simulink model "offlineDTOptim"  (R2019b)
settings: Solver=FixedStepAuto  StartTime=0.0  StopTime=tsim  FixedStep=1  MaxStep=1e-3  RelTol=1e-3  AbsTol=1e-3
PreLoadFcn:
  | coef = 220e-6; % Seebeck coefficient
  | R_int = 0.02; % Total electrical resistance
  | K = 1.5e-3; % Thermal conductance
  | T = 323.15; % Cold side temperature
  | 
  | 
StopFcn:
  | ee_addSimlogTimeStamp(bdroot)
values from neighbouring files (symbols this model uses):
  R = 3.3    [readSLDOData.m]
libraries: fl_lib x17, nesl_utility x10, ee_lib x5, simulink x2
CloseFcn:
  | try,close(h1_ee_peltier_device),end
  | clear h1_ee_peltier_device
  | 
  | clear simlog_ee_peltier_device
  | clear logsout_ee_peltier_device
  | clear COP_vec DT K R_int T coef j legend_data power simlog_Qc simlog_handles simlog_i simlog_v simout temp_cold_vec temp_hot temp_hot_vec
Description:
  | Use of Peltier Device as Thermoelectric Cooler
settings Model: OrderedModelArguments=off  Creator=The MathWorks, Inc.  LastModifiedBy=jairo
settings SolverCC: DecoupledContinuousIntegration=on
settings DataIOCC: SaveFormat=Array  ReturnWorkspaceOutputs=off  ReturnWorkspaceOutputsName=simout
settings OptimizationCC: LifeSpan=inf
settings DebuggingCC: UnderspecifiedInitializationDetection=Classic  MergeDetectMultiDrivingBlocksExec=none  SolverPrmCheckMsg=warning  FrameProcessingCompatibilityMsg=warning  StateNameClashWarn=warning  StrictBusMsg=ErrorOnBusTreatedAsVector  NonBusSignalsTreatedAsBus=error  SFUnexpectedBacktrackingDiag=warning  SFNoUnconditionalDefaultTransitionDiag=warning  ArithmeticOperatorsInVariantConditions=warning
settings HardwareCC: ProdBitPerPointer=32  ProdBitPerSizeT=32  ProdBitPerPtrDiffT=32  ProdLargestAtomicFloat=None  ProdIntDivRoundTo=Undefined  ProdEndianess=Unspecified  ProdWordSize=32  ProdHWDeviceType=32-bit Generic
settings ModelReferenceCC: PropagateSignalLabelsOutOfModel=off
settings SFSimCC: SimUseLocalCustomCode=off  CustomCodeUndefinedFunction=UseInterfaceOnly
settings RTWCC: RTWUseLocalCustomCode=off
settings GRTTargetCC: CodeReplacementLibrary=ANSI_C
settings SimscapeCC: SimscapeLogType=all  SimscapeLogSimulationStatistics=on  SimscapeLogName=simlog_ee_peltier_device  SimscapeLogDataHistory=10000

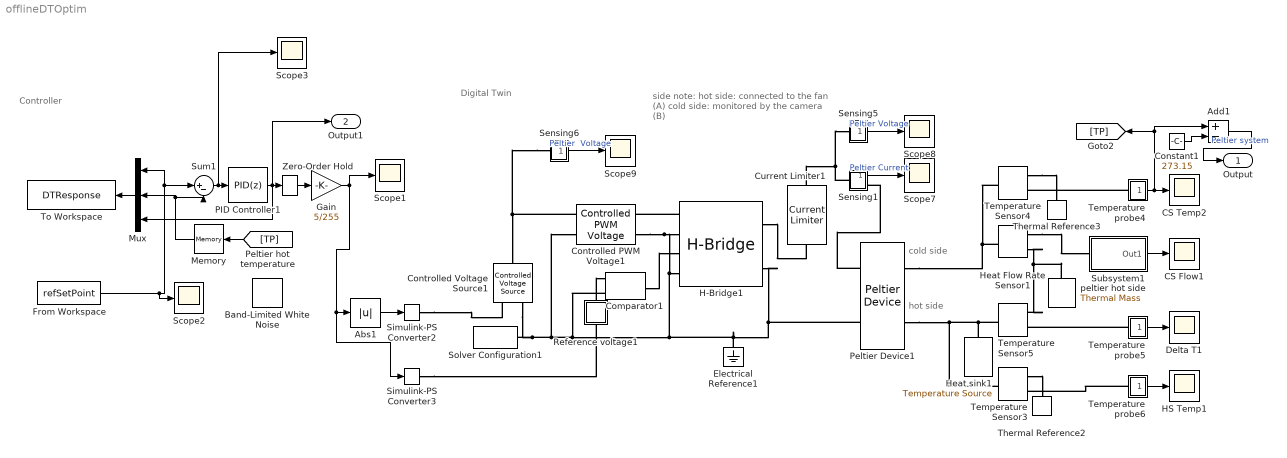
== system offlineDTOptim ==
  note: Digital Twin
  note: side note:
      |
      | hot side: connected to the fan (A)
      |
      | cold side: monitored by the camera (B)
  note: Controller
  note: cold side
  note: hot side
  Abs1 : Abs
  Add1 : Sum  Inputs=+-
  Band-Limited White Noise : simulink/Sources/Band-Limited White Noise  Cov=[0.005]  Ts=1  seed=[23341]
  CS Flow1 : Scope
  CS Temp2 : Scope
  Comparator1 : ee_lib/Integrated Circuits/Comparator  V_OS=5 mV  V_OL=0 V  V_OH=5 V  C_IN=0 pF  R_OUT=50 Ohm  Delay=0 s
      settings: SourceProductName=Simscape Electrical  SourceProductBaseCode=PS  InternalSimscapePortConfiguration="{\"Bottom\":[],\"Left\":[{\"id\":\"p\",\"label\":\"+\",\"type\":\"foundation.electrical.electrical\"},{\"id\":\"n\",\"label\":\"-\",\"type\":\"foundation.electrical.electrical\"}],\"Right\":[{\"id\":\"J\",\"label\":\"\",\"type\":\"foundation.electrical.electrical\"}],\"Top\":[]}"
  Constant1 : Constant  Value=273.15
  Controlled PWM Voltage1 : ee_lib/Integrated Circuits/Controlled PWM Voltage  F=4000 Hz  TD=0 s  pulse_width_offset=0 s  pulse_min=0 s  Vmin=0 V  Vmax=5 V  Vm=5 V  pwm_or_av=2  event_type=1  sample_time=5e-6 s  u_min=0  u_max=1
      settings: SourceProductName=Simscape Electrical
  Controlled Voltage Source1 : fl_lib/Electrical/Electrical Sources/Controlled Voltage Source
  Current Limiter1 : ee_lib/Semiconductors & Converters/Current Limiter  iLim=5 A  vLim=0.1 V  gLim=1e-3 1/Ohm  thermal_mass=100 J/K  initial_temperature=298.15 K
      settings: SourceProductName=Simscape Electrical  SourceProductBaseCode=PS  InternalSimscapePortConfiguration="{\"Bottom\":[],\"Left\":[{\"id\":\"p\",\"label\":\"+\",\"type\":\"foundation.electrical.electrical\"}],\"Right\":[{\"id\":\"n\",\"label\":\"-\",\"type\":\"foundation.electrical.electrical\"}],\"Top\":[]}"
  Delta T1 : Scope
  Electrical Reference1 : fl_lib/Electrical/Electrical Elements/Electrical Reference
  From Workspace : FromWorkspace  VariableName=refSetPoint  SampleTime=0
  Gain : Gain  Gain=5/255
  H-Bridge1 : ee_lib/Semiconductors & Converters/Converters/H-Bridge  supply_ports=ee.enum.supply_ports.hidesupply  Venable=2.5 V  Vmax=5 V  Vreverse=0.1 V  Vbrake=2.5 V  Vm=12 V  pwm_or_av=ee.enum.pwm_or_av.averaged  regenerative_braking_mode=ee.enum.converters.regenerative_braking_mode.always_enabled  discontinuous=ee.enum.current_profile.continuous  freewheeling_mode=ee.enum.converters.freewheeling_mode.one_switch_one_diode  Ron=0.1 Ohm  Don=0.1 Ohm  Goff=1e-6 S  Rload=3.38+0.1 Ohm  Lload=1e-5 H  F=4 kHz  thermal_mass=100 J/K  initial_temperature=298.15 K  Ron2=0.1 Ohm  Don2=0.05 Ohm  Tmeas=298.15 K  Tmeas2=398.15 K
      settings: SourceProductName=Simscape Electrical
  HS Temp1 : Scope
  Heat Flow Rate Sensor1 : fl_lib/Thermal/Thermal Sensors/Heat Flow Rate Sensor
      settings: SourceProductName=Simscape  SourceProductBaseCode=SS
  Heat sink1 : fl_lib/Thermal/Thermal Sources/Temperature Source  temperature=296 K
      settings: SourceProductName=Simscape
  Memory : Memory  InitialCondition=295
  Mux : Mux  Inputs=3
  PID Controller1 : simulink/Continuous/PID Controller  Controller=PID  Form=Parallel  TimeDomain=Discrete-time  SampleTime=1  IntegratorMethod=Forward Euler  FilterMethod=Forward Euler  ControllerParametersSource=internal  P=38.57  I=1.46877  D=6.66875  UseFilter=off  N=100  TunerSelectOption=Transfer Function Based (PID Tuner App)  InitialConditionSource=internal  InitialConditionForIntegrator=0  InitialConditionForFilter=0  DifferentiatorICPrevScaledInput=0  ExternalReset=none  TrackingMode=off  Kt=1  LimitOutput=on  UpperSaturationLimit=255  LowerSaturationLimit=-255  LinearizeAsGain=on  AntiWindupMode=back-calculation  Kb=1  POutMin=[]  POutMax=[]  IOutMin=[]  IOutMax=[]  DOutMin=[]  DOutMax=[]  NOutMin=[]  NOutMax=[]  SumOutMin=[]  SumOutMax=[]  SaturationOutMin=[]  SaturationOutMax=[]  PParamMin=[]  PParamMax=[]  IParamMin=[]  IParamMax=[]  DParamMin=[]  DParamMax=[]  NParamMin=[]  NParamMax=[]  KbParamMin=[]  KbParamMax=[]  KtParamMin=[]  KtParamMax=[]  KbOutMin=[]  KbOutMax=[]  KtOutMin=[]  KtOutMax=[]  IntegratorOutMin=[]  IntegratorOutMax=[]  FilterOutMin=[]  FilterOutMax=[]  SumI1OutMin=[]  SumI1OutMax=[]  SumI2OutMin=[]  SumI2OutMax=[]  SumI3OutMin=[]  SumI3OutMax=[]  SumI4OutMin=[]  SumI4OutMax=[]  SumDOutMin=[]  SumDOutMax=[]  DifferentiatorOutMin=[]  DifferentiatorOutMax=[]  FilterDiffOutCoefMin=[]  FilterDiffOutCoefMax=[]  ReciprocalOutMin=[]  ReciprocalOutMax=[]  SumDenOutMin=[]  SumDenOutMax=[]  SumNumOutMin=[]  SumNumOutMax=[]  DivideOutMin=[]  DivideOutMax=[]  IntegratorContinuousStateAttributes=''  IntegratorStateMustResolveToSignalObject=off  IntegratorRTWStateStorageClass=Auto  FilterContinuousStateAttributes=''  FilterStateMustResolveToSignalObject=off  FilterRTWStateStorageClass=Auto  ParallelPVariant=InternalParameters  IdealPVariant=Disabled  IVariant=InternalParameters  DVariant=InternalParameters  IntegratorVariant=Discrete  SatVariant=Enabled  AWVariant=BackCalculation  PCopyVariant=Disabled  TRVariant=Disabled  FdbkBlocksVariant=Forward  IdealPFdbkVariant=Disabled  SatFdbkVariant=Disabled  DerivativeFilterVariant=Differentiator  NVariant=Passthrough  NCopyVariant=Disabled_SignalSpec  FilterICVariant=InternalICsDifferentiator  IntegratorICVariant=InternalICs  ExternalResetVariant=Disabled  TRSumVariant=Passthrough  SumFdbkVariant=Disabled  SumVariant=Sum_PID
  Peltier Device1 : ee_lib/Sensors & Transducers/Peltier Device  alpha=alpha V/K  R=R Ohm  K=K W/K
      settings: SourceProductName=Simscape Electrical  SourceProductBaseCode=PS  InternalSimscapePortConfiguration="{\"Bottom\":[],\"Left\":[{\"id\":\"p\",\"label\":\"+\",\"type\":\"foundation.electrical.electrical\"},{\"id\":\"n\",\"label\":\"-\",\"type\":\"foundation.electrical.electrical\"}],\"Right\":[{\"id\":\"A\",\"label\":\"A\",\"type\":\"foundation.thermal.thermal\"},{\"id\":\"B\",\"label\":\"B\",\"type\":\"foundation.thermal.thermal\"}],\"Top\":[]}"
  Reference voltage1 : Subsystem
      mask Display: disp('Vr')
  Scope{1..3,7..9} (6 alike) : Scope
  Sensing1 : Subsystem
      mask Display: disp('A')
  Sensing5 : Subsystem
      mask Display: disp('V')
  Sensing6 : Subsystem
      mask Display: disp('V')
  Simulink-PS Converter2 : nesl_utility/Simulink-PS Converter  PhysicalDomain=network_engine_domain  SubClassName=ps_input  LeftPortType=input  RightPortType=output  PseudoPeriodic=off  Frequencies=[]  NoiseDistribution=none  NoiseParameters=[]  Unit=1  AffineConversion=off  FilteringAndDerivatives=provide  SimscapeFilterOrder=1  InputFilterTimeConstant=0.001  UdotUserProvided=0
  Simulink-PS Converter3 : nesl_utility/Simulink-PS Converter  PhysicalDomain=network_engine_domain  SubClassName=ps_input  LeftPortType=input  RightPortType=output  PseudoPeriodic=off  Frequencies=[]  NoiseDistribution=none  NoiseParameters=[]  Unit=1  AffineConversion=off  FilteringAndDerivatives=provide  SimscapeFilterOrder=1  InputFilterTimeConstant=0.001  UdotUserProvided=0
  Solver Configuration1 : nesl_utility/Solver Configuration  PhysicalDomain=network_engine_domain  SubClassName=solver  LeftPortType=input  RightPortType=generic  Tones=[]  Harmonics=[]  SimulateNoise=off  Profile=off  UseLocalSampling=off  EnableSwitchedLinearOptims=on  FrequencyDomain=off  UseCCode=off  RelTol=0.001  AbsTol=1e-06  MinStep=1e-09  ToWorkspace=off  RevertToSquareIcSolve=off  NumHomotopyIterations=100  PhasorMode=off  PhasorModeNumHarmonics=1  DoDC=off  ResidualTolerance=1e-09  UseLocalSolver=off  LocalSolverChoice=NE_BACKWARD_EULER_ADVANCER  LocalSolverSampleTime=0.001  DoFixedCost=off  MaxNonlinIter=3  MaxModeIter=2  LinearAlgebra=auto  EquationFormulation=NE_TIME_EF  DelaysMemoryBudget=1024  AutomaticFiltering=on  FilteringTimeConstant=0.001  PartitionStorageMethod=AS_NEEDED  PartitionMemoryBudget=1024  PartitionMethod=FAST
  Subsystem1 : Subsystem
      mask Display: disp('Heat flow')
  Sum1 : Sum  Inputs=|+-
  Temperature Sensor3 : fl_lib/Thermal/Thermal Sensors/Temperature Sensor
  Temperature Sensor4 : fl_lib/Thermal/Thermal Sensors/Temperature Sensor
  Temperature Sensor5 : fl_lib/Thermal/Thermal Sensors/Temperature Sensor
  Temperature probe4 : Subsystem
      mask Display: disp('T')
  Temperature probe5 : Subsystem
      mask Display: disp('T')
  Temperature probe6 : Subsystem
      mask Display: disp('T')
  Thermal Reference2 : fl_lib/Thermal/Thermal Elements/Thermal Reference
  Thermal Reference3 : fl_lib/Thermal/Thermal Elements/Thermal Reference
  To Workspace : ToWorkspace  VariableName=DTResponse  SaveFormat=Structure With Time  SampleTime=-1
  Zero-Order Hold : ZeroOrderHold
  peltier hot side : fl_lib/Thermal/Thermal Elements/Thermal Mass  mass=1 kg  sp_heat=C J/kg/K  T_specify=on  T_priority=High  T=296 K  T_nominal_specify=off  T_nominal_unit=K  T_nominal_value=1  Q_specify=off  Q_priority=Low  Q=0 W  Q_nominal_specify=off  Q_nominal_unit=W  Q_nominal_value=1
  Output : Outport
  Output1 : Outport  Port=2
  wires:
  From Workspace/1 -> Mux/1, Sum1/1, Scope2/1
  Sensing6/1(Out1) -> Scope9/1  "Peltier  Voltage"
  Sum1/1 -> Scope3/1, PID Controller1/1
  Temperature probe5/1(K) -> Delta T1/1
  Abs1/1 -> Simulink-PS Converter2/1
  Sensing5/1(Out1) -> Scope8/1  "Peltier Voltage"
  PID Controller1/1 -> Output1/1, Mux/3, Zero-Order Hold/1
  Sensing1/1(Out1) -> Scope7/1  "Peltier Current"
  Temperature probe6/1(K) -> HS Temp1/1
  Subsystem1/1(Out1) -> CS Flow1/1
  Gain/1 -> Scope1/1, Simulink-PS Converter3/1, Abs1/1
  Zero-Order Hold/1 -> Gain/1
  Temperature probe4/1(K) -> Add1/1, [TP], CS Temp2/1
  Constant1/1 -> Add1/2
  Add1/1 -> Output/1  "Peltier system"
  Mux/1 -> To Workspace/1
  [TP] -> Memory/1
  Memory/1 -> Sum1/2, Mux/2
  connections:
  H-Bridge1/LConn2 -- Comparator1/LConn2 -- Controlled Voltage Source1/RConn2 -- Solver Configuration1/RConn1 -- Controlled PWM Voltage1/LConn2 -- Electrical Reference1/LConn1 -- H-Bridge1/RConn2 -- Peltier Device1/LConn2 -- H-Bridge1/LConn4 -- Controlled PWM Voltage1/RConn2
  Sensing5/LConn1 -- Sensing1/LConn1 -- Current Limiter1/RConn1
  Temperature Sensor5/RConn1 -- Heat Flow Rate Sensor1/RConn2 -- peltier hot side/LConn1
  Sensing6/LConn1 -- Controlled PWM Voltage1/LConn1 -- Controlled Voltage Source1/LConn1
  Temperature Sensor4/LConn1 -- Heat Flow Rate Sensor1/LConn1 -- Peltier Device1/RConn1
  Temperature Sensor5/LConn1 -- Heat sink1/LConn1 -- Temperature Sensor3/LConn1 -- Peltier Device1/RConn2
  Reference voltage1/LConn1 -- Comparator1/LConn1
  Temperature probe5/LConn1 -- Temperature Sensor5/RConn2
  Peltier Device1/LConn1 -- Sensing1/RConn1
  Temperature Sensor4/RConn1 -- Thermal Reference3/LConn1
  Comparator1/RConn1 -- H-Bridge1/LConn3
  Temperature probe4/LConn1 -- Temperature Sensor4/RConn2
  H-Bridge1/RConn1 -- Current Limiter1/LConn1
  H-Bridge1/LConn1 -- Controlled PWM Voltage1/RConn1
  Heat Flow Rate Sensor1/RConn1 -- Subsystem1/LConn1
  Temperature probe6/LConn1 -- Temperature Sensor3/RConn2
  Temperature Sensor3/RConn1 -- Thermal Reference2/LConn1
  Simulink-PS Converter2/RConn1 -- Controlled Voltage Source1/RConn1
  Simulink-PS Converter3/RConn1 -- Reference voltage1/RConn1

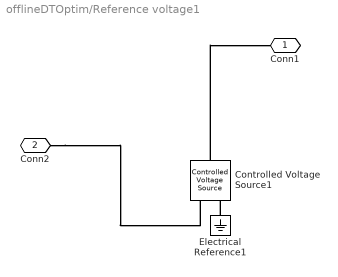
== system offlineDTOptim/Reference voltage1 ==
  Controlled Voltage Source1 : fl_lib/Electrical/Electrical Sources/Controlled Voltage Source
  Electrical Reference1 : fl_lib/Electrical/Electrical Elements/Electrical Reference
  Conn1 : PMIOPort  Side=Left
  Conn2 : PMIOPort  Port=2  Side=Right
  connections:
  Electrical Reference1/LConn1 -- Controlled Voltage Source1/RConn2
  Controlled Voltage Source1/LConn1 -- Conn1/RConn1
  Conn2/RConn1 -- Controlled Voltage Source1/RConn1

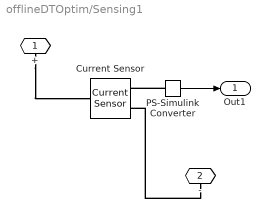
== system offlineDTOptim/Sensing1 ==
  Current Sensor : fl_lib/Electrical/Electrical Sensors/Current Sensor
  PS-Simulink Converter : nesl_utility/PS-Simulink Converter  PhysicalDomain=network_engine_domain  SubClassName=ps_output  LeftPortType=input  RightPortType=output  PseudoPeriodic=off  Frequencies=[]  Unit=inherit  AffineConversion=off
  + : PMIOPort  Side=Left
  - : PMIOPort  Port=2  Side=Right
  Out1 : Outport  VectorParamsAs1DForOutWhenUnconnected=off
  wires:
  PS-Simulink Converter/1 -> Out1/1
  connections:
  +/RConn1 -- Current Sensor/LConn1
  PS-Simulink Converter/LConn1 -- Current Sensor/RConn1
  -/RConn1 -- Current Sensor/RConn2

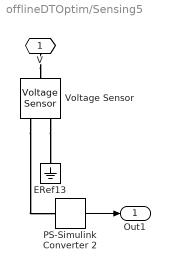
== system offlineDTOptim/Sensing5 ==
  ERef13 : fl_lib/Electrical/Electrical Elements/Electrical Reference
  PS-Simulink Converter 2 : nesl_utility/PS-Simulink Converter  PhysicalDomain=network_engine_domain  SubClassName=ps_output  LeftPortType=input  RightPortType=output  PseudoPeriodic=off  Frequencies=[]  Unit=V  AffineConversion=off
  Voltage Sensor : fl_lib/Electrical/Electrical Sensors/Voltage Sensor
  V : PMIOPort  Side=Left
  Out1 : Outport  VectorParamsAs1DForOutWhenUnconnected=off
  wires:
  PS-Simulink Converter 2/1 -> Out1/1
  connections:
  V/RConn1 -- Voltage Sensor/LConn1
  Voltage Sensor/RConn2 -- ERef13/LConn1
  Voltage Sensor/RConn1 -- PS-Simulink Converter 2/LConn1

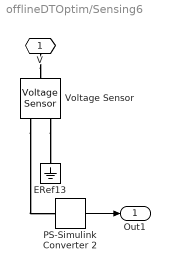
== system offlineDTOptim/Sensing6 ==
  ERef13 : fl_lib/Electrical/Electrical Elements/Electrical Reference
  PS-Simulink Converter 2 : nesl_utility/PS-Simulink Converter  PhysicalDomain=network_engine_domain  SubClassName=ps_output  LeftPortType=input  RightPortType=output  PseudoPeriodic=off  Frequencies=[]  Unit=V  AffineConversion=off
  Voltage Sensor : fl_lib/Electrical/Electrical Sensors/Voltage Sensor
  V : PMIOPort  Side=Left
  Out1 : Outport  VectorParamsAs1DForOutWhenUnconnected=off
  wires:
  PS-Simulink Converter 2/1 -> Out1/1
  connections:
  V/RConn1 -- Voltage Sensor/LConn1
  Voltage Sensor/RConn2 -- ERef13/LConn1
  Voltage Sensor/RConn1 -- PS-Simulink Converter 2/LConn1

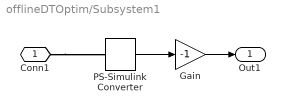
== system offlineDTOptim/Subsystem1 ==
  Gain : Gain  Gain=-1
  PS-Simulink Converter : nesl_utility/PS-Simulink Converter  PhysicalDomain=network_engine_domain  SubClassName=ps_output  LeftPortType=input  RightPortType=output  PseudoPeriodic=off  Frequencies=[]  Unit=J/s  AffineConversion=off
  Conn1 : PMIOPort  Side=Left
  Out1 : Outport  VectorParamsAs1DForOutWhenUnconnected=off
  wires:
  Gain/1 -> Out1/1
  PS-Simulink Converter/1 -> Gain/1
  connections:
  Conn1/RConn1 -- PS-Simulink Converter/LConn1

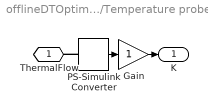
== system offlineDTOptim/Temperature probe4 ==
  Gain : Gain
  PS-Simulink Converter : nesl_utility/PS-Simulink Converter  PhysicalDomain=network_engine_domain  SubClassName=ps_output  LeftPortType=input  RightPortType=output  PseudoPeriodic=off  Frequencies=[]  Unit=K  AffineConversion=off
  ThermalFlow : PMIOPort  Side=Left
  K : Outport
  wires:
  PS-Simulink Converter/1 -> Gain/1
  Gain/1 -> K/1
  connections:
  PS-Simulink Converter/LConn1 -- ThermalFlow/RConn1

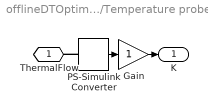
== system offlineDTOptim/Temperature probe5 ==
  Gain : Gain
  PS-Simulink Converter : nesl_utility/PS-Simulink Converter  PhysicalDomain=network_engine_domain  SubClassName=ps_output  LeftPortType=input  RightPortType=output  PseudoPeriodic=off  Frequencies=[]  Unit=K  AffineConversion=off
  ThermalFlow : PMIOPort  Side=Left
  K : Outport
  wires:
  PS-Simulink Converter/1 -> Gain/1
  Gain/1 -> K/1
  connections:
  PS-Simulink Converter/LConn1 -- ThermalFlow/RConn1

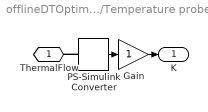
== system offlineDTOptim/Temperature probe6 ==
  Gain : Gain
  PS-Simulink Converter : nesl_utility/PS-Simulink Converter  PhysicalDomain=network_engine_domain  SubClassName=ps_output  LeftPortType=input  RightPortType=output  PseudoPeriodic=off  Frequencies=[]  Unit=K  AffineConversion=off
  ThermalFlow : PMIOPort  Side=Left
  K : Outport
  wires:
  PS-Simulink Converter/1 -> Gain/1
  Gain/1 -> K/1
  connections:
  PS-Simulink Converter/LConn1 -- ThermalFlow/RConn1
